simulink model "swingBalanceFuzzy"  (Simulink 8.1)
settings: Solver=ode45  StartTime=0.0  StopTime=20  RelTol=1e-3
StopFcn:
  | subplot(2,1,1);
  | plot(Data.time,Data.signals(1,1).values,'-r','LineWidth',1.5)
  | legend('alpha');
  | grid;
  | ylabel('alpha [rad]]');
  | title('Pendulum');
  | %subplot(2,1,2);
  | %plot(Data.time,Data.signals(1,2).values,'-c','LineWidth',2.5)
  | %hold on;
  | %plot(Data.time,Data.signals(1,3).values,'--b','LineWidth',2)
  | %grid;
  | %legend('y','y dot');
  | %ylabel('Position of Ball [m]');
  | subplot(2,1,2);
  | plot(Data.time,Data.signals(1,3).values,'-g','LineWidth',1.5)
  | legend('theta');
  | grid;
  | ylabel('theta [rad]');
libraries: fuzblock x2
settings Model: Creator=ThanhNhan  LastModifiedBy=ThanhNhan
settings DataIOCC: SignalLoggingSaveFormat=Dataset
settings OptimizationCC: ExpressionDepthLimit=128
settings DebuggingCC: FcnCallInpInsideContextMsg=EnableAllAsError
settings GRTTargetCC: CombineOutputUpdateFcns=on  GRTInterface=off

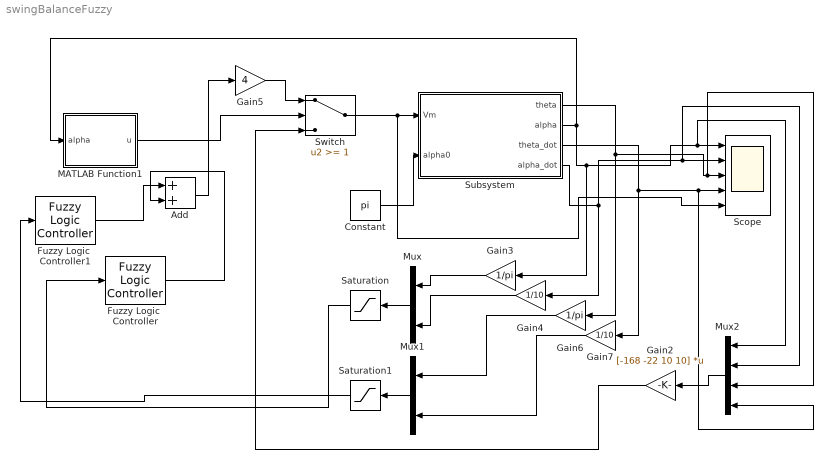
== system swingBalanceFuzzy ==
  Add : Sum
  Constant : Constant  Value=pi
  Fuzzy Logic  Controller : fuzblock/Fuzzy Logic  Controller  fis='SimpleFLC2input.fis'
  Fuzzy Logic  Controller1 : fuzblock/Fuzzy Logic  Controller  fis='SimpleFLC2input.fis'
  Gain2 : Gain  Gain=[-168 -22 10 10]  Multiplication=Matrix(K*u)
  Gain3 : Gain  Gain=1/pi
  Gain4 : Gain  Gain=1/10
  Gain5 : Gain  Gain=4
  Gain6 : Gain  Gain=1/pi
  Gain7 : Gain  Gain=1/10
  MATLAB Function1 : MATLAB Function  TreatAsAtomicUnit=on
  Mux : Mux  Inputs=2
  Mux1 : Mux  Inputs=2
  Mux2 : Mux
  Saturation : Saturate  UpperLimit=1  LowerLimit=-1
  Saturation1 : Saturate  UpperLimit=1  LowerLimit=-1
  Scope : Scope  NumInputPorts=5
      settings: TimeRange=30  YMin=0~-20~-1700~-105~-24  YMax=13~20~-600~-70~-10  SaveName=Data
  Subsystem : Subsystem  mask{Jeq=0.0095842, g=9.81, m=0.09, L=0.15, r=0.224, Beq=0.0144, eta=0.69, Km=0.084026, Kt=0.084039, Rm=0.59, Jm=0.001}
      mask prompts: Jeq "Momen quán tính tuong duong"; g "Gia toc trong truong"; m "Khoi luong con lac"; L "Chieu dai con lac"; r "Chieu dài cánh tay"; Beq "He so can tuong duong"; eta "Hieu suat dong co"; Km "Hang so suc dien dong"; Kt "Hang so momen"; Rm "Dien tro phan ung"; Jm "Momen quan tinh"
  Switch : Switch  Threshold=1
  wires:
  Subsystem/1(theta) -> Mux2/3, Scope/3, Gain6/1
  Switch/1 -> Scope/5, Subsystem/1(Vm)
  Subsystem/2(alpha) -> Mux2/1, Scope/1, Gain3/1, MATLAB Function1/1(alpha)
  MATLAB Function1/1(u) -> Switch/2
  Mux/1 -> Saturation/1
  Fuzzy Logic  Controller/1 -> Add/2
  Saturation/1 -> Fuzzy Logic  Controller/1
  Gain3/1 -> Mux/1
  Gain4/1 -> Mux/2
  Gain6/1 -> Mux1/1
  Gain7/1 -> Mux1/2
  Constant/1 -> Subsystem/2(alpha0)
  Mux1/1 -> Saturation1/1
  Saturation1/1 -> Fuzzy Logic  Controller1/1
  Fuzzy Logic  Controller1/1 -> Add/1
  Add/1 -> Gain5/1
  Gain5/1 -> Switch/1
  Mux2/1 -> Gain2/1
  Subsystem/4(alpha_dot) -> Mux2/2, Scope/2, Gain4/1
  Subsystem/3(theta_dot) -> Mux2/4, Scope/4, Gain7/1
  Gain2/1 -> Switch/3

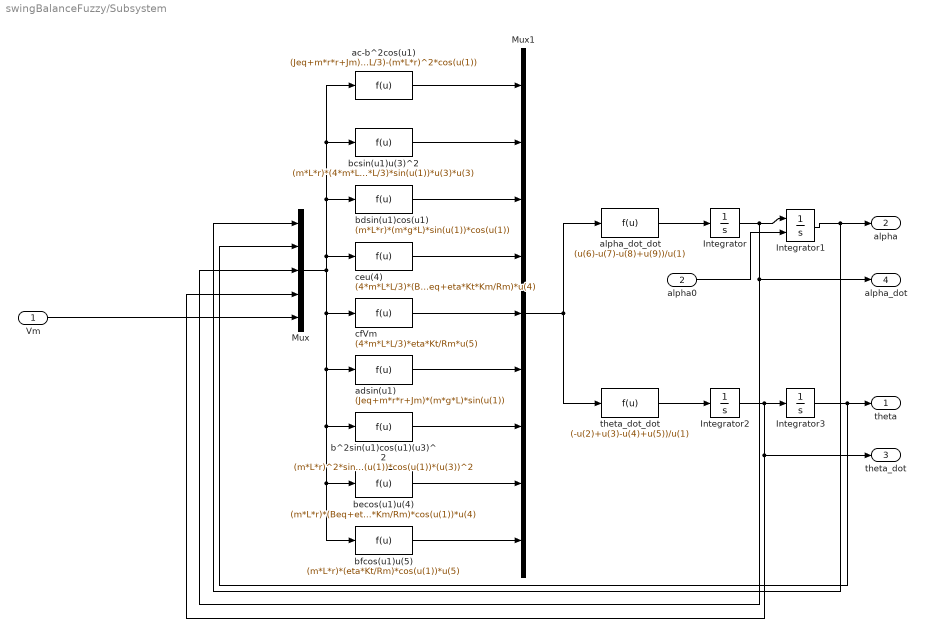
== system swingBalanceFuzzy/Subsystem ==
  Vm : Inport
  alpha0 : Inport  Port=2
  Integrator : Integrator  UpperSaturationLimit=pi/18  LowerSaturationLimit=-pi/18
  Integrator1 : Integrator  InitialConditionSource=external  InitialCondition=pi  UpperSaturationLimit=pi/18  LowerSaturationLimit=-pi/18
  Integrator2 : Integrator
  Integrator3 : Integrator  UpperSaturationLimit=2  LowerSaturationLimit=-2
  Mux : Mux  Inputs=5
  Mux1 : Mux  Inputs=9
  ac-b^2cos(u1) : Fcn  Expr=(Jeq+m*r*r+Jm)*(4*m*L*L/3)-(m*L*r)^2*cos(u(1))
  adsin(u1) : Fcn  Expr=(Jeq+m*r*r+Jm)*(m*g*L)*sin(u(1))
  alpha_dot_dot : Fcn  Expr=(u(6)-u(7)-u(8)+u(9))/u(1)
  b^2sin(u1)cos(u1)(u3)^2 : Fcn  Expr=(m*L*r)^2*sin(u(1))*cos(u(1))*(u(3))^2
  bcsin(u1)u(3)^2 : Fcn  Expr=(m*L*r)*(4*m*L*L/3)*sin(u(1))*u(3)*u(3)
  bdsin(u1)cos(u1) : Fcn  Expr=(m*L*r)*(m*g*L)*sin(u(1))*cos(u(1))
  becos(u1)u(4) : Fcn  Expr=(m*L*r)*(Beq+eta*Kt*Km/Rm)*cos(u(1))*u(4)
  bfcos(u1)u(5) : Fcn  Expr=(m*L*r)*(eta*Kt/Rm)*cos(u(1))*u(5)
  ceu(4) : Fcn  Expr=(4*m*L*L/3)*(Beq+eta*Kt*Km/Rm)*u(4)
  cfVm : Fcn  Expr=(4*m*L*L/3)*eta*Kt/Rm*u(5)
  theta_dot_dot : Fcn  Expr=(-u(2)+u(3)-u(4)+u(5))/u(1)
  theta : Outport
  alpha : Outport  Port=2
  theta_dot : Outport  Port=3
  alpha_dot : Outport  Port=4
  wires:
  alpha_dot_dot/1 -> Integrator/1
  Integrator/1 -> Mux/3, alpha_dot/1, Integrator1/1
  theta_dot_dot/1 -> Integrator2/1
  Integrator1/1 -> Mux/1, alpha/1
  Integrator3/1 -> Mux/2, theta/1
  ac-b^2cos(u1)/1 -> Mux1/1
  bcsin(u1)u(3)^2/1 -> Mux1/2
  bdsin(u1)cos(u1)/1 -> Mux1/3
  ceu(4)/1 -> Mux1/4
  cfVm/1 -> Mux1/5
  adsin(u1)/1 -> Mux1/6
  b^2sin(u1)cos(u1)(u3)^2/1 -> Mux1/7
  becos(u1)u(4)/1 -> Mux1/8
  bfcos(u1)u(5)/1 -> Mux1/9
  Mux1/1 -> theta_dot_dot/1, alpha_dot_dot/1
  Mux/1 -> ceu(4)/1, bdsin(u1)cos(u1)/1, bcsin(u1)u(3)^2/1, ac-b^2cos(u1)/1, bfcos(u1)u(5)/1, becos(u1)u(4)/1, b^2sin(u1)cos(u1)(u3)^2/1, adsin(u1)/1, cfVm/1
  Integrator2/1 -> Mux/4, theta_dot/1, Integrator3/1
  Vm/1 -> Mux/5
  alpha0/1 -> Integrator1/2

== matlab function MATLAB Function1 ==
  data: u output double; alpha input double
function u = fcn(alpha)
%#codegen

if (alpha<pi/10)||(alpha>19*pi/10)
    u=0;
else u=1;
end

%y = u;
